simulink model "task_2"  (R2021a)
settings: Solver=VariableStepAuto  StartTime=0.0  StopTime=50.0  RelTol=1e-3
values from neighbouring files (symbols this model uses):
  A = [0,0,1,0 ... (first row only)    [task1.m]    (also in task2.m)
  B = [0;0;1/mc;1/(L*mc)]    [task1.m]    (also in task2.m)
settings Model: Creator=hp  LastModifiedBy=hp

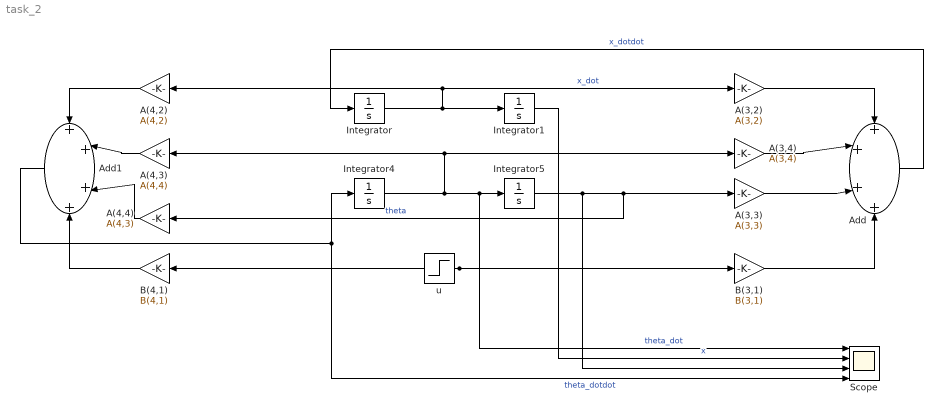
== system task_2 ==
  A(3,2) : Gain  Gain=A(3,2)
  A(3,3) : Gain  Gain=A(3,3)
  A(3,4) : Gain  Gain=A(3,4)
  A(4,2) : Gain  Gain=A(4,2)
  A(4,3) : Gain  Gain=A(4,4)
  A(4,4) : Gain  Gain=A(4,3)
  Add : Sum  Inputs=++++
  Add1 : Sum  Inputs=++++
  B(3,1) : Gain  Gain=B(3,1)
  B(4,1) : Gain  Gain=B(4,1)
  Integrator{,1,4..5} (4 alike) : Integrator
  Scope : Scope  NumInputPorts=4
  u : Step  SampleTime=0
  wires:
  Integrator/1 -> Integrator1/1, A(3,2)/1, A(4,2)/1  "x_dot"
  Add/1 -> Integrator/1  "x_dotdot"
  Integrator1/1 -> Scope/2  "x"
  Integrator4/1 -> A(3,4)/1, A(4,3)/1, Scope/1, Integrator5/1  "theta_dot"
  Integrator5/1 -> Scope/3, A(3,3)/1, A(4,4)/1  "theta"
  u/1 -> B(3,1)/1, B(4,1)/1
  A(3,2)/1 -> Add/1
  A(3,4)/1 -> Add/2
  A(3,3)/1 -> Add/3
  B(3,1)/1 -> Add/4
  A(4,2)/1 -> Add1/1
  A(4,3)/1 -> Add1/2
  A(4,4)/1 -> Add1/3
  B(4,1)/1 -> Add1/4
  Add1/1 -> Integrator4/1, Scope/4  "theta_dotdot"
